simulink model "DAB_3phase_final"  (R2022b)
settings: Solver=ode23t  StartTime=0.0  StopTime=1/100000*10000  MaxStep=1/100000  RelTol=1e-3  AbsTol=1e-3
StartFcn:
  | tic
StopFcn:
  | toc
undefined symbols (not defined in the file): Vdc, Vth
libraries: nesl_utility x24, fl_lib x21, ee_lib x13, simulink x6, slpidlib x1
settings Model: SimulationMode=accelerator  Creator=jvansick  LastModifiedBy=jvansick
settings SolverCC: ExtrapolationOrder=1  ZeroCrossAlgorithm=Adaptive  ODENIntegrationMethod=ode14x
settings DebuggingCC: UnconnectedInputMsg=warning  UnconnectedOutputMsg=warning  UnconnectedLineMsg=warning
settings ModelReferenceCC: EnableRefExpFcnMdlSchedulingChecks=on
settings RTWCC: DLArmComputeVersion=19.05

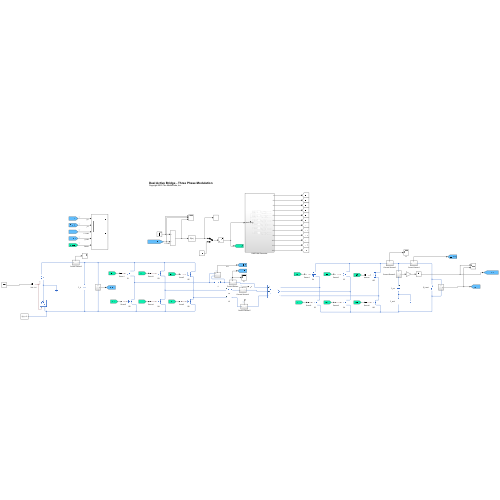
[thumbnail: Simulink's stored preview of the top-level diagram]
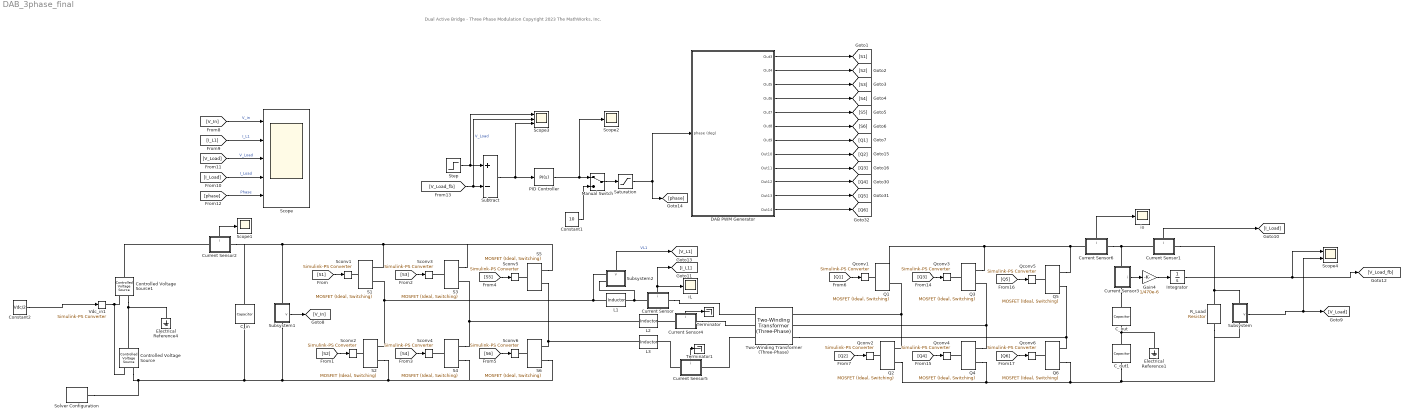
== system DAB_3phase_final ==
  note: Dual Active Bridge - Three Phase Modulation
      | Copyright 2023 The MathWorks, Inc.
  C_in : fl_lib/Electrical/Electrical Elements/Capacitor  c=220e-6 F  r=1e-6 Ohm  g=0 1/Ohm  i_specify=off  i_priority=None  i=0 A  i_nominal_specify=off  i_nominal_unit=A  i_nominal_value=1  v_specify=off  v_priority=None  v=0 V  v_nominal_specify=off  v_nominal_unit=V  v_nominal_value=1  vc_specify=on  vc_priority=High  vc=Vdc V  vc_nominal_specify=off  vc_nominal_unit=V  vc_nominal_value=1
  C_out : fl_lib/Electrical/Electrical Elements/Capacitor  c=(470e-6)*2 F  r=0 Ohm  g=0 1/Ohm  i_specify=off  i_priority=None  i=0 A  i_nominal_specify=off  i_nominal_unit=A  i_nominal_value=1  v_specify=off  v_priority=None  v=0 V  v_nominal_specify=off  v_nominal_unit=V  v_nominal_value=1  vc_specify=on  vc_priority=High  vc=200 V  vc_nominal_specify=off  vc_nominal_unit=V  vc_nominal_value=1
  C_out1 : fl_lib/Electrical/Electrical Elements/Capacitor  c=(470e-6)*2 F  r=0 Ohm  g=0 1/Ohm  i_specify=off  i_priority=None  i=0 A  i_nominal_specify=off  i_nominal_unit=A  i_nominal_value=1  v_specify=off  v_priority=None  v=0 V  v_nominal_specify=off  v_nominal_unit=V  v_nominal_value=1  vc_specify=on  vc_priority=High  vc=200 V  vc_nominal_specify=off  vc_nominal_unit=V  vc_nominal_value=1
  Constant1 : Constant  Value=10  SampleTime=-1
  Constant2 : Constant  Value=Vdc/2
  Controlled Voltage Source : fl_lib/Electrical/Electrical Sources/Controlled Voltage Source
  Controlled Voltage Source1 : fl_lib/Electrical/Electrical Sources/Controlled Voltage Source
  Current Sensor : Subsystem
      settings: PortSchema="{\"entries\":[{\"content\":{\"sides\":[{\"content\":{\"connectorIds\":[\"LConn1\"]},\"type\":\"ConnectorPlacement.EquallySpacedRectSide\",\"uuid\":\"e9388151-e471-4783-81c5-5134e1313d7c\"},{\"content\":{\"connectorIds\":[\"RConn1\"],\"side\":\"RIGHT\"},\"type\":\"ConnectorPlacement.EquallySpacedRectSide\",\"uuid\":\"bcb23f28-0826-4736-ab91-150a314eb643\"},{\"content\":{\"connectorIds\":[\"Out1\"],\"side\":\"TOP\"},\"type\":\"ConnectorPlacement.EquallySpacedRectSide\",\"uuid\":\"e1937689-3337-4922-a316-f56c73fb0974\"}]},\"type\":\"ConnectorPlacement.EquallySpacedConnector\",\"uuid\":\"dc34a384-5aa5-46fc-88a5-47651899efae\"}],\"packageUris\":[\"http://schema.mathworks.com/mf0/Connector/R2020b\"],\"version\":\"1.0\"}"
  Current Sensor1 : Subsystem
      settings: PortSchema="{\"entries\":[{\"content\":{\"sides\":[{\"content\":{\"connectorIds\":[\"LConn1\"]},\"type\":\"ConnectorPlacement.EquallySpacedRectSide\",\"uuid\":\"e9388151-e471-4783-81c5-5134e1313d7c\"},{\"content\":{\"connectorIds\":[\"RConn1\"],\"side\":\"RIGHT\"},\"type\":\"ConnectorPlacement.EquallySpacedRectSide\",\"uuid\":\"bcb23f28-0826-4736-ab91-150a314eb643\"},{\"content\":{\"connectorIds\":[\"Out1\"],\"side\":\"TOP\"},\"type\":\"ConnectorPlacement.EquallySpacedRectSide\",\"uuid\":\"e1937689-3337-4922-a316-f56c73fb0974\"}]},\"type\":\"ConnectorPlacement.EquallySpacedConnector\",\"uuid\":\"dc34a384-5aa5-46fc-88a5-47651899efae\"}],\"packageUris\":[\"http://schema.mathworks.com/mf0/Connector/R2020b\"],\"version\":\"1.0\"}"
  Current Sensor2 : Subsystem
      settings: PortSchema="{\"entries\":[{\"content\":{\"sides\":[{\"content\":{\"connectorIds\":[\"LConn1\"]},\"type\":\"ConnectorPlacement.EquallySpacedRectSide\",\"uuid\":\"e9388151-e471-4783-81c5-5134e1313d7c\"},{\"content\":{\"connectorIds\":[\"RConn1\"],\"side\":\"RIGHT\"},\"type\":\"ConnectorPlacement.EquallySpacedRectSide\",\"uuid\":\"bcb23f28-0826-4736-ab91-150a314eb643\"},{\"content\":{\"connectorIds\":[\"Out1\"],\"side\":\"TOP\"},\"type\":\"ConnectorPlacement.EquallySpacedRectSide\",\"uuid\":\"e1937689-3337-4922-a316-f56c73fb0974\"}]},\"type\":\"ConnectorPlacement.EquallySpacedConnector\",\"uuid\":\"dc34a384-5aa5-46fc-88a5-47651899efae\"}],\"packageUris\":[\"http://schema.mathworks.com/mf0/Connector/R2020b\"],\"version\":\"1.0\"}"
  Current Sensor3 : Subsystem
      settings: PortSchema="{\"entries\":[{\"content\":{\"sides\":[{\"content\":{\"connectorIds\":[\"LConn1\"]},\"type\":\"ConnectorPlacement.EquallySpacedRectSide\",\"uuid\":\"e9388151-e471-4783-81c5-5134e1313d7c\"},{\"content\":{\"connectorIds\":[\"RConn1\"],\"side\":\"RIGHT\"},\"type\":\"ConnectorPlacement.EquallySpacedRectSide\",\"uuid\":\"bcb23f28-0826-4736-ab91-150a314eb643\"},{\"content\":{\"connectorIds\":[\"Out1\"],\"side\":\"TOP\"},\"type\":\"ConnectorPlacement.EquallySpacedRectSide\",\"uuid\":\"e1937689-3337-4922-a316-f56c73fb0974\"}]},\"type\":\"ConnectorPlacement.EquallySpacedConnector\",\"uuid\":\"dc34a384-5aa5-46fc-88a5-47651899efae\"}],\"packageUris\":[\"http://schema.mathworks.com/mf0/Connector/R2020b\"],\"version\":\"1.0\"}"
  Current Sensor4 : Subsystem
      settings: PortSchema="{\"entries\":[{\"content\":{\"sides\":[{\"content\":{\"connectorIds\":[\"LConn1\"]},\"type\":\"ConnectorPlacement.EquallySpacedRectSide\",\"uuid\":\"e9388151-e471-4783-81c5-5134e1313d7c\"},{\"content\":{\"connectorIds\":[\"RConn1\"],\"side\":\"RIGHT\"},\"type\":\"ConnectorPlacement.EquallySpacedRectSide\",\"uuid\":\"bcb23f28-0826-4736-ab91-150a314eb643\"},{\"content\":{\"connectorIds\":[\"Out1\"],\"side\":\"TOP\"},\"type\":\"ConnectorPlacement.EquallySpacedRectSide\",\"uuid\":\"e1937689-3337-4922-a316-f56c73fb0974\"}]},\"type\":\"ConnectorPlacement.EquallySpacedConnector\",\"uuid\":\"dc34a384-5aa5-46fc-88a5-47651899efae\"}],\"packageUris\":[\"http://schema.mathworks.com/mf0/Connector/R2020b\"],\"version\":\"1.0\"}"
  Current Sensor5 : Subsystem
      settings: PortSchema="{\"entries\":[{\"content\":{\"sides\":[{\"content\":{\"connectorIds\":[\"LConn1\"]},\"type\":\"ConnectorPlacement.EquallySpacedRectSide\",\"uuid\":\"e9388151-e471-4783-81c5-5134e1313d7c\"},{\"content\":{\"connectorIds\":[\"RConn1\"],\"side\":\"RIGHT\"},\"type\":\"ConnectorPlacement.EquallySpacedRectSide\",\"uuid\":\"bcb23f28-0826-4736-ab91-150a314eb643\"},{\"content\":{\"connectorIds\":[\"Out1\"],\"side\":\"TOP\"},\"type\":\"ConnectorPlacement.EquallySpacedRectSide\",\"uuid\":\"e1937689-3337-4922-a316-f56c73fb0974\"}]},\"type\":\"ConnectorPlacement.EquallySpacedConnector\",\"uuid\":\"dc34a384-5aa5-46fc-88a5-47651899efae\"}],\"packageUris\":[\"http://schema.mathworks.com/mf0/Connector/R2020b\"],\"version\":\"1.0\"}"
  Current Sensor6 : Subsystem
      settings: PortSchema="{\"entries\":[{\"content\":{\"sides\":[{\"content\":{\"connectorIds\":[\"LConn1\"]},\"type\":\"ConnectorPlacement.EquallySpacedRectSide\",\"uuid\":\"e9388151-e471-4783-81c5-5134e1313d7c\"},{\"content\":{\"connectorIds\":[\"RConn1\"],\"side\":\"RIGHT\"},\"type\":\"ConnectorPlacement.EquallySpacedRectSide\",\"uuid\":\"bcb23f28-0826-4736-ab91-150a314eb643\"},{\"content\":{\"connectorIds\":[\"Out1\"],\"side\":\"TOP\"},\"type\":\"ConnectorPlacement.EquallySpacedRectSide\",\"uuid\":\"e1937689-3337-4922-a316-f56c73fb0974\"}]},\"type\":\"ConnectorPlacement.EquallySpacedConnector\",\"uuid\":\"dc34a384-5aa5-46fc-88a5-47651899efae\"}],\"packageUris\":[\"http://schema.mathworks.com/mf0/Connector/R2020b\"],\"version\":\"1.0\"}"
  DAB PWM Generator : Subsystem
  Electrical Reference1 : fl_lib/Electrical/Electrical Elements/Electrical Reference
  Electrical Reference4 : fl_lib/Electrical/Electrical Elements/Electrical Reference
  Gain4 : Gain  Gain=1/470e-6
  Integrator : Integrator  InitialCondition=400
  L1 : fl_lib/Electrical/Electrical Elements/Inductor  l=36e-6 H  r=0.01 Ohm  g=1e-6 1/Ohm  i_specify=off  i_priority=None  i=0 A  i_nominal_specify=off  i_nominal_unit=A  i_nominal_value=1  v_specify=off  v_priority=None  v=0 V  v_nominal_specify=off  v_nominal_unit=V  v_nominal_value=1  i_L_specify=off  i_L_priority=High  i_L=0 A  i_L_nominal_specify=off  i_L_nominal_unit=A  i_L_nominal_value=1
  L2 : fl_lib/Electrical/Electrical Elements/Inductor  l=36e-6 H  r=0.01 Ohm  g=1e-6 1/Ohm  i_specify=off  i_priority=None  i=0 A  i_nominal_specify=off  i_nominal_unit=A  i_nominal_value=1  v_specify=off  v_priority=None  v=0 V  v_nominal_specify=off  v_nominal_unit=V  v_nominal_value=1  i_L_specify=off  i_L_priority=High  i_L=0 A  i_L_nominal_specify=off  i_L_nominal_unit=A  i_L_nominal_value=1
  L3 : fl_lib/Electrical/Electrical Elements/Inductor  l=36e-6 H  r=0.01 Ohm  g=1e-6 1/Ohm  i_specify=off  i_priority=None  i=0 A  i_nominal_specify=off  i_nominal_unit=A  i_nominal_value=1  v_specify=off  v_priority=None  v=0 V  v_nominal_specify=off  v_nominal_unit=V  v_nominal_value=1  i_L_specify=off  i_L_priority=High  i_L=0 A  i_L_nominal_specify=off  i_L_nominal_unit=A  i_L_nominal_value=1
  Manual Switch : ManualSwitch
  PID Controller : slpidlib/PID Controller  Controller=PI  Form=Parallel  TimeDomain=Continuous-time  UseExternalTs=off  SampleTime=-1  IntegratorMethod=Forward Euler  FilterMethod=Forward Euler  ControllerParametersSource=internal  P=0.3  I=60  UseKiTs=off  D=0  N=100  UseFilter=on  TunerSelectOption=Transfer Function Based (PID Tuner App)  InitialConditionSource=internal  InitialConditionForIntegrator=0  InitialConditionForFilter=0  DifferentiatorICPrevScaledInput=0  ExternalReset=none  TrackingMode=off  Kt=1  LimitOutput=off  SatLimitsSource=internal  UpperSaturationLimit=inf  LowerSaturationLimit=-inf  LinearizeAsGain=on  AntiWindupMode=none  Kb=1  LimitIntegrator=off  UpperIntegratorSaturationLimit=inf  LowerIntegratorSaturationLimit=-inf  POutMin=[]  POutMax=[]  IOutMin=[]  IOutMax=[]  DOutMin=[]  DOutMax=[]  NOutMin=[]  NOutMax=[]  SumOutMin=[]  SumOutMax=[]  SaturationOutMin=[]  SaturationOutMax=[]  PParamMin=[]  PParamMax=[]  IParamMin=[]  IParamMax=[]  DParamMin=[]  DParamMax=[]  NParamMin=[]  NParamMax=[]  KbParamMin=[]  KbParamMax=[]  KtParamMin=[]  KtParamMax=[]  KbOutMin=[]  KbOutMax=[]  KtOutMin=[]  KtOutMax=[]  IntegratorOutMin=[]  IntegratorOutMax=[]  FilterOutMin=[]  FilterOutMax=[]  SumI1OutMin=[]  SumI1OutMax=[]  SumI2OutMin=[]  SumI2OutMax=[]  SumI3OutMin=[]  SumI3OutMax=[]  SumI4OutMin=[]  SumI4OutMax=[]  SumDOutMin=[]  SumDOutMax=[]  DifferentiatorOutMin=[]  DifferentiatorOutMax=[]  FilterDiffOutCoefMin=[]  FilterDiffOutCoefMax=[]  ReciprocalOutMin=[]  ReciprocalOutMax=[]  SumDenOutMin=[]  SumDenOutMax=[]  SumNumOutMin=[]  SumNumOutMax=[]  DivideOutMin=[]  DivideOutMax=[]  UdiffTsProdOutMin=[]  UdiffTsProdOutMax=[]  NTsProdOutMin=[]  NTsProdOutMax=[]  UintegralTsProdOutMin=[]  UintegralTsProdOutMax=[]  UngainTsProdOutMin=[]  UngainTsProdOutMax=[]  ClampingZeroOutDataTypeStr=Inherit: Inherit via back propagation  ClampingZeroOutMin=[]  ClampingZeroOutMax=[]  FilterDenConstantOutDataTypeStr=Inherit: Inherit via back propagation  FilterDenConstantOutMin=[]  FilterDenConstantOutMax=[]  PCopyOutDataTypeStr=Inherit: Inherit via back propagation  PCopyOutMin=[]  PCopyOutMax=[]  NCopyOutDataTypeStr=Inherit: Inherit via back propagation  NCopyOutMin=[]  NCopyOutMax=[]  IntegratorContinuousStateAttributes=''  IntegratorStateMustResolveToSignalObject=off  IntegratorRTWStateStorageClass=Auto  FilterContinuousStateAttributes=''  FilterStateMustResolveToSignalObject=off  FilterRTWStateStorageClass=Auto  ParallelPVariant=InternalParameters  IdealPVariant=Disabled  IVariant=InternalParameters  DVariant=Disabled  IntegratorVariant=Continuous  SatVariant=Disabled  AWVariant=Passthrough  PCopyVariant=Disabled  TRVariant=Disabled  FdbkBlocksVariant=Forward  IdealPFdbkVariant=Disabled  SatFdbkVariant=Disabled  DerivativeFilterVariant=Disabled  NVariant=Disabled  NCopyVariant=Disabled_SignalSpec  FilterICVariant=Disabled  IntegratorICVariant=InternalICs  ExternalResetVariant=Disabled  TRSumVariant=Passthrough  SumFdbkVariant=Disabled  SumVariant=Sum_PI  TsampFilterVariant=InternalTs  TsampNgainVariant=Passthrough  TsampIntegralVariant=Passthrough  ExternalSaturationOutDataTypeStr=Inherit: Same as second input
  Q{1..6} (6 alike) : ee_lib/Semiconductors & Converters/MOSFET (Ideal, Switching)  port_option=ee.enum.controlport.ps  Rds=R_ds Ohm  Goff=1e-5 1/Ohm  Vth=Vth V  diode_param=2  diode_Vf=0.8 V  diode_Ron=0.001 Ohm  diode_Goff=1e-5 1/Ohm  diode_C=50e-9 F  diode_iRM=-235 A  diode_iF=300 A  diode_idot=-50 A/us  diode_trr_param=1  diode_trr_factor=3  diode_trr=15 us  diode_Qrr=1500 s*uA  ids_specify=off  ids_priority=None  ids=0 A  ids_nominal_specify=off  ids_nominal_unit=A  ids_nominal_value=1  vds_specify=off  vds_priority=None  vds=0 V  vds_nominal_specify=off  vds_nominal_unit=V  vds_nominal_value=1  vgs_specify=off  vgs_priority=None  vgs=0 V  vgs_nominal_specify=off  vgs_nominal_unit=V  vgs_nominal_value=1  thermal_loss_option=ee.enum.converters.thermalLossOption.constantvalues  Von_data=[0, 1.8, 3.2, 6, 10, 16; 0, 2, 5.5, 9.5, 15, 25] V  Tj=[298.15, 448.15] K  Iout_data=[0, 20, 40, 60, 80, 100] A  Eon_data=[0, 55.04, 124.57, 235.53, 362.12; 0, 71.25, 161.25, 304.88, 468.75] * 1e-6 J  Eoff_data=[0, 18, 30, 56.1, 76.5; 0, 22.5, 37.5, 70.13, 95.63] * 1e-6 J  Tj_loss=[298.15, 448.15] K  Iout_data_loss=[0, 10, 20, 30, 40] A  Eon_scalar=22.86e-3 J  Eoff_scalar=17.14e-3 J  Voff=300 V  Iout_scalar=600 A  diodeModelType=ee.enum.converters.diodeModelType.pwl  diodeTableType=ee.enum.diode.tableType.IfMat  diode_IfMat=[.07, .12, .19, 1.75, 4.24, 7.32, 11.2; .16, .3, .72, 2.14, 4.02, 6.35, 9.12] A  diode_VfMat=[.9, 1.15, 1.25, 1.5, 1.75, 2.17, 2.6, 2.85; .58, .68, .75, 1.1, 1.38, 1.77, 2.27, 2.7] V  diode_TjVec=[25, 125] degC  diode_VfVec=[.5, .7, .9, 1.3, 1.7, 2.1, 2.5] V  diode_IfVec=[.1, .2, .5, 1, 2, 4, 7, 10] A  diode_Vr=-600 V  diode_Ls=150 nH  diode_Erec=0.03 J  thermal_network_parameterization=ee.enum.thermalNetworkTopology.external  Rth=[.03, .2] K/W  Rth_Cauer=[.03, .1, .2] K/W  Rth_Foster=[.03, .2] K/W  thermal_mass_parameterization=ee.enum.thermalNetwork.timeconstant  thermal_mass=[3, 25] J/K  thermal_mass_Cauer=[3, 10, 25] J/K  thermal_mass_Foster=[33, 50] J/K  thermal_time_constant=[.1, 5] s  thermal_time_constant_Cauer=[.1, 1, 5] s  thermal_time_constant_Foster=[1, 10] s  thermal_mass_initial_temperatures=[25, 25] degC  thermal_mass_initial_temperatures_Cauer=[25, 25, 25] degC  junction_thermal_mass=0.1 J/K  Tvec_initial_Foster=[25, 25, 25, 25] degC  no_thermal_network=0  junction_temperature_specify=off  junction_temperature_priority=None  junction_temperature=25 degC  junction_temperature_nominal_specify=off  junction_temperature_nominal_unit=degC  junction_temperature_nominal_value=1  Qj_specify=off  Qj_priority=None  Qj=0 W  Qj_nominal_specify=off  Qj_nominal_unit=W  Qj_nominal_value=1
  Qconv{1..6} (6 alike) : nesl_utility/Simulink-PS Converter  PhysicalDomain=network_engine_domain  SubClassName=ps_input  LeftPortType=input  RightPortType=output  PseudoPeriodic=off  Frequencies=[]  NoiseDistribution=none  NoiseParameters=[]  Unit=1  AffineConversion=off  FilteringAndDerivatives=provide  SimscapeFilterOrder=1  InputFilterTimeConstant=0.001  UdotUserProvided=0
  R_Load : fl_lib/Electrical/Electrical Elements/Resistor  R=26 Ohm  i_specify=off  i_priority=None  i=0 A  i_nominal_specify=off  i_nominal_unit=A  i_nominal_value=1  v_specify=off  v_priority=None  v=0 V  v_nominal_specify=off  v_nominal_unit=V  v_nominal_value=1
  S{1..6} (6 alike) : ee_lib/Semiconductors & Converters/MOSFET (Ideal, Switching)  port_option=ee.enum.controlport.ps  Rds=R_ds Ohm  Goff=1e-5 1/Ohm  Vth=Vth V  diode_param=2  diode_Vf=0.8 V  diode_Ron=0.001 Ohm  diode_Goff=1e-5 1/Ohm  diode_C=50e-9 F  diode_iRM=-235 A  diode_iF=300 A  diode_idot=-50 A/us  diode_trr_param=1  diode_trr_factor=3  diode_trr=15 us  diode_Qrr=1500 s*uA  ids_specify=off  ids_priority=None  ids=0 A  ids_nominal_specify=off  ids_nominal_unit=A  ids_nominal_value=1  vds_specify=off  vds_priority=None  vds=0 V  vds_nominal_specify=off  vds_nominal_unit=V  vds_nominal_value=1  vgs_specify=off  vgs_priority=None  vgs=0 V  vgs_nominal_specify=off  vgs_nominal_unit=V  vgs_nominal_value=1  thermal_loss_option=ee.enum.converters.thermalLossOption.constantvalues  Von_data=[0, 1.8, 3.2, 6, 10, 16; 0, 2, 5.5, 9.5, 15, 25] V  Tj=[298.15, 448.15] K  Iout_data=[0, 20, 40, 60, 80, 100] A  Eon_data=[0, 55.04, 124.57, 235.53, 362.12; 0, 71.25, 161.25, 304.88, 468.75] * 1e-6 J  Eoff_data=[0, 18, 30, 56.1, 76.5; 0, 22.5, 37.5, 70.13, 95.63] * 1e-6 J  Tj_loss=[298.15, 448.15] K  Iout_data_loss=[0, 10, 20, 30, 40] A  Eon_scalar=22.86e-3 J  Eoff_scalar=17.14e-3 J  Voff=300 V  Iout_scalar=600 A  diodeModelType=ee.enum.converters.diodeModelType.pwl  diodeTableType=ee.enum.diode.tableType.IfMat  diode_IfMat=[.07, .12, .19, 1.75, 4.24, 7.32, 11.2; .16, .3, .72, 2.14, 4.02, 6.35, 9.12] A  diode_VfMat=[.9, 1.15, 1.25, 1.5, 1.75, 2.17, 2.6, 2.85; .58, .68, .75, 1.1, 1.38, 1.77, 2.27, 2.7] V  diode_TjVec=[25, 125] degC  diode_VfVec=[.5, .7, .9, 1.3, 1.7, 2.1, 2.5] V  diode_IfVec=[.1, .2, .5, 1, 2, 4, 7, 10] A  diode_Vr=-600 V  diode_Ls=150 nH  diode_Erec=0.03 J  thermal_network_parameterization=ee.enum.thermalNetworkTopology.external  Rth=[.03, .2] K/W  Rth_Cauer=[.03, .1, .2] K/W  Rth_Foster=[.03, .2] K/W  thermal_mass_parameterization=ee.enum.thermalNetwork.timeconstant  thermal_mass=[3, 25] J/K  thermal_mass_Cauer=[3, 10, 25] J/K  thermal_mass_Foster=[33, 50] J/K  thermal_time_constant=[.1, 5] s  thermal_time_constant_Cauer=[.1, 1, 5] s  thermal_time_constant_Foster=[1, 10] s  thermal_mass_initial_temperatures=[25, 25] degC  thermal_mass_initial_temperatures_Cauer=[25, 25, 25] degC  junction_thermal_mass=0.1 J/K  Tvec_initial_Foster=[25, 25, 25, 25] degC  no_thermal_network=0  junction_temperature_specify=off  junction_temperature_priority=None  junction_temperature=25 degC  junction_temperature_nominal_specify=off  junction_temperature_nominal_unit=degC  junction_temperature_nominal_value=1  Qj_specify=off  Qj_priority=None  Qj=0 W  Qj_nominal_specify=off  Qj_nominal_unit=W  Qj_nominal_value=1
  Saturation : Saturate  UpperLimit=180  LowerLimit=0
  Sconv{1..6} (6 alike) : nesl_utility/Simulink-PS Converter  PhysicalDomain=network_engine_domain  SubClassName=ps_input  LeftPortType=input  RightPortType=output  PseudoPeriodic=off  Frequencies=[]  NoiseDistribution=none  NoiseParameters=[]  Unit=1  AffineConversion=off  FilteringAndDerivatives=provide  SimscapeFilterOrder=1  InputFilterTimeConstant=0.001  UdotUserProvided=0
  Scope : Scope  NumInputPorts=5
  Scope1 : Scope
  Scope2 : Scope
  Scope3 : Scope  NumInputPorts=3
  Scope4 : Scope  NumInputPorts=2
  Solver Configuration : nesl_utility/Solver Configuration  PhysicalDomain=network_engine_domain  SubClassName=solver  LeftPortType=input  RightPortType=generic  Tones=[]  Harmonics=[]  SimulateNoise=off  Profile=off  UseLocalSampling=off  EnableSwitchedLinearOptims=on  FrequencyDomain=off  UseCCode=off  RelTol=0.001  AbsTol=1e-06  MinStep=1e-09  ToWorkspace=off  RevertToSquareIcSolve=off  NumHomotopyIterations=100  PhasorMode=off  PhasorModeNumHarmonics=1  ConsistencySolver=NEWTON_FTOL  IndexReductionMethod=DerivativeReplacement  DoDC=off  ResidualTolerance=1e-09  ConsistencyTolSource=GLOBAL  ConsistencyAbsTol=0.001  ConsistencyRelTol=0.001  ConsistencyTolFactor=0.001  UseLocalSolver=off  LocalSolverChoice=NE_BACKWARD_EULER_ADVANCER  ResolveIndetEquations=on  FunctionEvalNumThread=1  LocalSolverSampleTime=1/100000/100  DoFixedCost=off  MaxNonlinIter=3  MaxModeIter=2  ComputeImpulses=off  ImpulseIterations=2  LinearAlgebra=auto  LinearAlgebraNumThread=0  EquationFormulation=NE_TIME_EF  DelaysMemoryBudget=1024  AutomaticFiltering=on  FilteringTimeConstant=0.001  PartitionStorageMethod=AS_NEEDED  PartitionMemoryBudget=1024  PartitionMethod=ROBUST
  Step : Step  Time=1/100000*10000/2  Before=400  After=500  SampleTime=0
  Subsystem : Subsystem
      settings: PortSchema="{\"entries\":[{\"content\":{\"sides\":[{\"content\":{\"connectorIds\":[\"LConn1\"]},\"type\":\"ConnectorPlacement.EquallySpacedRectSide\",\"uuid\":\"e9388151-e471-4783-81c5-5134e1313d7c\"},{\"content\":{\"connectorIds\":[\"RConn1\"],\"side\":\"RIGHT\"},\"type\":\"ConnectorPlacement.EquallySpacedRectSide\",\"uuid\":\"bcb23f28-0826-4736-ab91-150a314eb643\"},{\"content\":{\"connectorIds\":[\"Out1\"],\"side\":\"TOP\"},\"type\":\"ConnectorPlacement.EquallySpacedRectSide\",\"uuid\":\"e1937689-3337-4922-a316-f56c73fb0974\"}]},\"type\":\"ConnectorPlacement.EquallySpacedConnector\",\"uuid\":\"dc34a384-5aa5-46fc-88a5-47651899efae\"}],\"packageUris\":[\"http://schema.mathworks.com/mf0/Connector/R2020b\"],\"version\":\"1.0\"}"
  Subsystem1 : Subsystem
      settings: PortSchema="{\"entries\":[{\"content\":{\"sides\":[{\"content\":{\"connectorIds\":[\"LConn1\"]},\"type\":\"ConnectorPlacement.EquallySpacedRectSide\",\"uuid\":\"e9388151-e471-4783-81c5-5134e1313d7c\"},{\"content\":{\"connectorIds\":[\"RConn1\"],\"side\":\"RIGHT\"},\"type\":\"ConnectorPlacement.EquallySpacedRectSide\",\"uuid\":\"bcb23f28-0826-4736-ab91-150a314eb643\"},{\"content\":{\"connectorIds\":[\"Out1\"],\"side\":\"TOP\"},\"type\":\"ConnectorPlacement.EquallySpacedRectSide\",\"uuid\":\"e1937689-3337-4922-a316-f56c73fb0974\"}]},\"type\":\"ConnectorPlacement.EquallySpacedConnector\",\"uuid\":\"dc34a384-5aa5-46fc-88a5-47651899efae\"}],\"packageUris\":[\"http://schema.mathworks.com/mf0/Connector/R2020b\"],\"version\":\"1.0\"}"
  Subsystem2 : Subsystem
      settings: PortSchema="{\"entries\":[{\"content\":{\"sides\":[{\"content\":{\"connectorIds\":[\"LConn1\",\"LConn2\"]},\"type\":\"ConnectorPlacement.EquallySpacedRectSide\",\"uuid\":\"e9388151-e471-4783-81c5-5134e1313d7c\"},{\"content\":{\"connectorIds\":[],\"side\":\"RIGHT\"},\"type\":\"ConnectorPlacement.EquallySpacedRectSide\",\"uuid\":\"bcb23f28-0826-4736-ab91-150a314eb643\"},{\"content\":{\"connectorIds\":[\"Out1\"],\"side\":\"TOP\"},\"type\":\"ConnectorPlacement.EquallySpacedRectSide\",\"uuid\":\"e1937689-3337-4922-a316-f56c73fb0974\"}]},\"type\":\"ConnectorPlacement.EquallySpacedConnector\",\"uuid\":\"dc34a384-5aa5-46fc-88a5-47651899efae\"}],\"packageUris\":[\"http://schema.mathworks.com/mf0/Connector/R2020b\"],\"version\":\"1.0\"}"
  Subtract : Sum  Inputs=+-
  Terminator : Terminator
  Terminator1 : Terminator
  Two-Winding Transformer (Three-Phase) : ee_lib/Passive/Transformers/Two-Winding Transformer (Three-Phase)  SRated=25e3 A*V  FRated=100000 Hz  Winding1Connection=ee.enum.windingconnection.Yg  VRated1=800 V  Winding2Connection=ee.enum.windingconnection.Yg  VRated2=500 V  CoreType=ee.enum.coretype.threelimb  pu_Rw1=0.01  pu_Rw2=0.01  leakage_reactance_option=ee.enum.transformer_leakage.exclude  pu_Xl1=0.05  pu_Xl2=0.05  magnetizing_resistance_option=ee.enum.transformer_magnetizingResistance.exclude  pu_Rm=500  magnetizing_reactance_option=ee.enum.transformer_magnetizingReactance.exclude  saturation_option=ee.enum.transformer_saturation.exclude  pu_Xm=500  current_data=[0, .002, 1, 2]  magnetic_flux_data=[0, 1.2, 1.5, 1.51]  pu_X0=0.5  i1_specify=off  i1_priority=None  i1=[0, 0, 0] A  i1_nominal_specify=off  i1_nominal_unit=A  i1_nominal_value=1  i2_specify=off  i2_priority=None  i2=[0, 0, 0] A  i2_nominal_specify=off  i2_nominal_unit=A  i2_nominal_value=1  phi_specify=off  phi_priority=None  phi=[0, 0, 0]  phi_nominal_specify=off  phi_nominal_unit=1  phi_nominal_value=1  power_dissipated_specify=off  power_dissipated_priority=None  power_dissipated=0 W  power_dissipated_nominal_specify=off  power_dissipated_nominal_unit=W  power_dissipated_nominal_value=1
      settings: InternalSimscapePortConfiguration="{\"Bottom\":[],\"Left\":[{\"id\":\"a1\",\"label\":\"a1\",\"type\":\"foundation.electrical.electrical\"},{\"id\":\"b1\",\"label\":\"b1\",\"type\":\"foundation.electrical.electrical\"},{\"id\":\"c1\",\"label\":\"c1\",\"type\":\"foundation.electrical.electrical\"}],\"Right\":[{\"id\":\"a2\",\"label\":\"a2\",\"type\":\"foundation.electrical.electrical\"},{\"id\":\"b2\",\"label\":\"b2\",\"type\":\"foundation.electrical.electrical\"},{\"id\":\"c2\",\"label\":\"c2\",\"type\":\"foundation.electrical.electrical\"}],\"Top\":[]}"
  Vdc_in1 : nesl_utility/Simulink-PS Converter  PhysicalDomain=network_engine_domain  SubClassName=ps_input  LeftPortType=input  RightPortType=output  PseudoPeriodic=off  Frequencies=[]  NoiseDistribution=none  NoiseParameters=[]  Unit=1  AffineConversion=off  FilteringAndDerivatives=provide  SimscapeFilterOrder=1  InputFilterTimeConstant=0.001  UdotUserProvided=0
  iL : Scope
  io : Scope
  wires:
  [S1] -> Sconv1/1
  [S2] -> Sconv2/1
  [S3] -> Sconv3/1
  [S4] -> Sconv4/1
  Subsystem1/1(v) -> [V_In]
  Subsystem/1(v) -> Scope4/2, [V_Load]
  Current Sensor1/1(i) -> [I_Load]
  Current Sensor/1(i) -> [I_L1], iL/1
  [V_In] -> Scope/1  "V_in"
  [I_L1] -> Scope/2  "I_L1"
  [I_Load] -> Scope/4  "I_Load"
  [V_Load] -> Scope/3  "V_Load"
  Current Sensor2/1(i) -> Scope1/1
  Current Sensor3/1(i) -> Gain4/1
  Integrator/1 -> Scope4/1, [V_Load_fb]
  Subsystem2/1(v) -> [V_L1]  "VL1"
  [phase] -> Scope/5  "Phase"
  [S6] -> Sconv6/1
  [S5] -> Sconv5/1
  [Q5] -> Qconv5/1
  [Q6] -> Qconv6/1
  [Q3] -> Qconv3/1
  [Q1] -> Qconv1/1
  [Q4] -> Qconv4/1
  [Q2] -> Qconv2/1
  Subtract/1 -> Scope3/3, PID Controller/1
  [V_Load_fb] -> Scope3/2, Subtract/2  "V_Load"
  Step/1 -> Scope3/1, Subtract/1
  Saturation/1 -> [phase], DAB PWM Generator/1(phase (deg))
  Current Sensor4/1(i) -> Terminator/1
  DAB PWM Generator/1(Out3) -> [S1]
  DAB PWM Generator/2(Out4) -> [S2]
  DAB PWM Generator/3(Out5) -> [S3]
  DAB PWM Generator/4(Out6) -> [S4]
  DAB PWM Generator/5(Out7) -> [S5]
  DAB PWM Generator/6(Out8) -> [S6]
  Current Sensor5/1(i) -> Terminator1/1
  DAB PWM Generator/7(Out9) -> [Q1]
  DAB PWM Generator/8(Out10) -> [Q2]
  DAB PWM Generator/9(Out11) -> [Q3]
  DAB PWM Generator/10(Out12) -> [Q4]
  DAB PWM Generator/11(Out13) -> [Q5]
  DAB PWM Generator/12(Out14) -> [Q6]
  Current Sensor6/1(i) -> io/1
  PID Controller/1 -> Scope2/1, Manual Switch/1
  Manual Switch/1 -> Saturation/1
  Constant1/1 -> Manual Switch/2
  Constant2/1 -> Vdc_in1/1
  Gain4/1 -> Integrator/1
  connections:
  Subsystem1/LConn1 -- Current Sensor2/RConn1 -- C_in/LConn1 -- S5/RConn1 -- S3/RConn1 -- S1/RConn1
  Controlled Voltage Source/RConn2 -- Solver Configuration/RConn1 -- Subsystem1/RConn1 -- S6/RConn2 -- S4/RConn2 -- S2/RConn2 -- C_in/RConn1
  S2/LConn1 -- Sconv2/RConn1
  Sconv1/RConn1 -- S1/LConn1
  S3/LConn1 -- Sconv3/RConn1
  S4/LConn1 -- Sconv4/RConn1
  Subsystem2/LConn1 -- S1/RConn2 -- S2/RConn1 -- L1/LConn1
  S4/RConn1 -- L2/LConn1 -- S3/RConn2
  R_Load/LConn1 -- Current Sensor1/RConn1 -- Subsystem/LConn1
  Current Sensor/LConn1 -- Subsystem2/LConn2 -- L1/RConn1
  Current Sensor3/RConn1 -- C_out/LConn1
  S5/RConn2 -- L3/LConn1 -- S6/RConn1
  S6/LConn1 -- Sconv6/RConn1
  S5/LConn1 -- Sconv5/RConn1
  Subsystem/RConn1 -- R_Load/RConn1 -- C_out1/RConn1 -- Q2/RConn2 -- Q4/RConn2 -- Q6/RConn2
  Current Sensor3/LConn1 -- Current Sensor6/RConn1 -- Current Sensor1/LConn1
  Q6/LConn1 -- Qconv6/RConn1
  Q3/LConn1 -- Qconv3/RConn1
  Q5/RConn2 -- Q6/RConn1 -- Two-Winding Transformer (Three-Phase)/RConn3
  Q2/RConn1 -- Q1/RConn2 -- Two-Winding Transformer (Three-Phase)/RConn1
  Q2/LConn1 -- Qconv2/RConn1
  Q4/LConn1 -- Qconv4/RConn1
  Q5/LConn1 -- Qconv5/RConn1
  Q4/RConn1 -- Q3/RConn2 -- Two-Winding Transformer (Three-Phase)/RConn2
  Qconv1/RConn1 -- Q1/LConn1
  Current Sensor4/LConn1 -- L2/RConn1
  Current Sensor5/LConn1 -- L3/RConn1
  Two-Winding Transformer (Three-Phase)/LConn3 -- Current Sensor5/RConn1
  Q5/RConn1 -- Current Sensor6/LConn1 -- Q1/RConn1 -- Q3/RConn1
  C_out1/LConn1 -- Electrical Reference1/LConn1 -- C_out/RConn1
  Vdc_in1/RConn1 -- Controlled Voltage Source1/RConn1 -- Controlled Voltage Source/RConn1
  Current Sensor2/LConn1 -- Controlled Voltage Source1/LConn1
  Controlled Voltage Source1/RConn2 -- Electrical Reference4/LConn1 -- Controlled Voltage Source/LConn1
  Current Sensor4/RConn1 -- Two-Winding Transformer (Three-Phase)/LConn2
  Current Sensor/RConn1 -- Two-Winding Transformer (Three-Phase)/LConn1

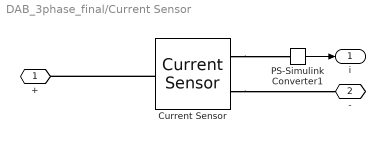
== system DAB_3phase_final/Current Sensor ==
  Current Sensor : fl_lib/Electrical/Electrical Sensors/Current Sensor
  PS-Simulink Converter1 : nesl_utility/PS-Simulink Converter  PhysicalDomain=network_engine_domain  SubClassName=ps_output  LeftPortType=input  RightPortType=output  PseudoPeriodic=off  Frequencies=[]  VectorFormat=1-D array  Unit=inherit  AffineConversion=off
  + : PMIOPort  Side=Left
  - : PMIOPort  Port=2  Side=Right
  i : Outport
  wires:
  PS-Simulink Converter1/1 -> i/1
  connections:
  Current Sensor/RConn1 -- PS-Simulink Converter1/LConn1
  Current Sensor/LConn1 -- +/RConn1
  Current Sensor/RConn2 -- -/RConn1

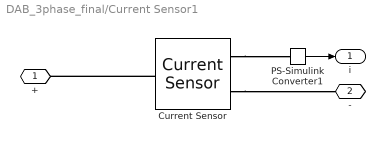
== system DAB_3phase_final/Current Sensor1 ==
  Current Sensor : fl_lib/Electrical/Electrical Sensors/Current Sensor
  PS-Simulink Converter1 : nesl_utility/PS-Simulink Converter  PhysicalDomain=network_engine_domain  SubClassName=ps_output  LeftPortType=input  RightPortType=output  PseudoPeriodic=off  Frequencies=[]  VectorFormat=1-D array  Unit=inherit  AffineConversion=off
  + : PMIOPort  Side=Left
  - : PMIOPort  Port=2  Side=Right
  i : Outport
  wires:
  PS-Simulink Converter1/1 -> i/1
  connections:
  Current Sensor/RConn2 -- -/RConn1
  Current Sensor/LConn1 -- +/RConn1
  Current Sensor/RConn1 -- PS-Simulink Converter1/LConn1

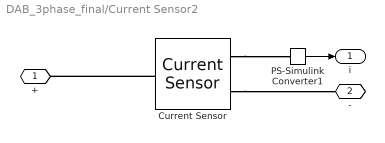
== system DAB_3phase_final/Current Sensor2 ==
  Current Sensor : fl_lib/Electrical/Electrical Sensors/Current Sensor
  PS-Simulink Converter1 : nesl_utility/PS-Simulink Converter  PhysicalDomain=network_engine_domain  SubClassName=ps_output  LeftPortType=input  RightPortType=output  PseudoPeriodic=off  Frequencies=[]  VectorFormat=1-D array  Unit=inherit  AffineConversion=off
  + : PMIOPort  Side=Left
  - : PMIOPort  Port=2  Side=Right
  i : Outport
  wires:
  PS-Simulink Converter1/1 -> i/1
  connections:
  Current Sensor/RConn2 -- -/RConn1
  Current Sensor/LConn1 -- +/RConn1
  Current Sensor/RConn1 -- PS-Simulink Converter1/LConn1

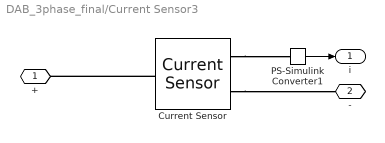
== system DAB_3phase_final/Current Sensor3 ==
  Current Sensor : fl_lib/Electrical/Electrical Sensors/Current Sensor
  PS-Simulink Converter1 : nesl_utility/PS-Simulink Converter  PhysicalDomain=network_engine_domain  SubClassName=ps_output  LeftPortType=input  RightPortType=output  PseudoPeriodic=off  Frequencies=[]  VectorFormat=1-D array  Unit=inherit  AffineConversion=off
  + : PMIOPort  Side=Left
  - : PMIOPort  Port=2  Side=Right
  i : Outport
  wires:
  PS-Simulink Converter1/1 -> i/1
  connections:
  Current Sensor/RConn1 -- PS-Simulink Converter1/LConn1
  Current Sensor/LConn1 -- +/RConn1
  Current Sensor/RConn2 -- -/RConn1

== system DAB_3phase_final/Current Sensor4 ==
  Current Sensor : fl_lib/Electrical/Electrical Sensors/Current Sensor
  PS-Simulink Converter1 : nesl_utility/PS-Simulink Converter  PhysicalDomain=network_engine_domain  SubClassName=ps_output  LeftPortType=input  RightPortType=output  PseudoPeriodic=off  Frequencies=[]  VectorFormat=1-D array  Unit=inherit  AffineConversion=off
  + : PMIOPort  Side=Left
  - : PMIOPort  Port=2  Side=Right
  i : Outport
  wires:
  PS-Simulink Converter1/1 -> i/1
  connections:
  Current Sensor/RConn1 -- PS-Simulink Converter1/LConn1
  Current Sensor/LConn1 -- +/RConn1
  Current Sensor/RConn2 -- -/RConn1

== system DAB_3phase_final/Current Sensor5 ==
  Current Sensor : fl_lib/Electrical/Electrical Sensors/Current Sensor
  PS-Simulink Converter1 : nesl_utility/PS-Simulink Converter  PhysicalDomain=network_engine_domain  SubClassName=ps_output  LeftPortType=input  RightPortType=output  PseudoPeriodic=off  Frequencies=[]  VectorFormat=1-D array  Unit=inherit  AffineConversion=off
  + : PMIOPort  Side=Left
  - : PMIOPort  Port=2  Side=Right
  i : Outport
  wires:
  PS-Simulink Converter1/1 -> i/1
  connections:
  Current Sensor/RConn1 -- PS-Simulink Converter1/LConn1
  Current Sensor/LConn1 -- +/RConn1
  Current Sensor/RConn2 -- -/RConn1

== system DAB_3phase_final/Current Sensor6 ==
  Current Sensor : fl_lib/Electrical/Electrical Sensors/Current Sensor
  PS-Simulink Converter1 : nesl_utility/PS-Simulink Converter  PhysicalDomain=network_engine_domain  SubClassName=ps_output  LeftPortType=input  RightPortType=output  PseudoPeriodic=off  Frequencies=[]  VectorFormat=1-D array  Unit=inherit  AffineConversion=off
  + : PMIOPort  Side=Left
  - : PMIOPort  Port=2  Side=Right
  i : Outport
  wires:
  PS-Simulink Converter1/1 -> i/1
  connections:
  Current Sensor/RConn1 -- PS-Simulink Converter1/LConn1
  Current Sensor/LConn1 -- +/RConn1
  Current Sensor/RConn2 -- -/RConn1

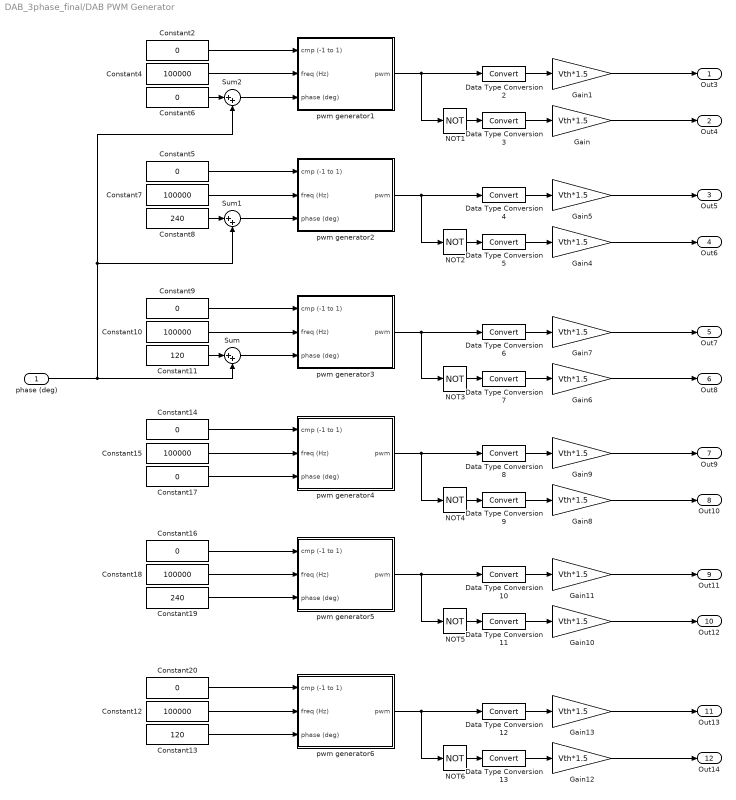
== system DAB_3phase_final/DAB PWM Generator ==
  phase (deg) : Inport
  Constant{4,7,10,12,15,18} (6 alike) : Constant  Value=100000
  Constant11 : Constant  Value=120
  Constant13 : Constant  Value=120
  Constant{2,5..6,9,14,16..17,20} (8 alike) : Constant  Value=0
  Constant19 : Constant  Value=240
  Constant8 : Constant  Value=240
  Data Type Conversion{2..13} (12 alike) : DataTypeConversion  SaturateOnIntegerOverflow=off  RndMeth=Floor
  Gain{,1,4..13} (12 alike) : Gain  Gain=Vth*1.5
  NOT{1..6} (6 alike) : Logic  Operator=NOT  IconShape=distinctive  AllPortsSameDT=off  OutDataTypeStr=boolean
  Sum : Sum  Inputs=|++
  Sum1 : Sum  Inputs=|++
  Sum2 : Sum  Inputs=|++
  pwm generator1 : Subsystem
  pwm generator2 : Subsystem
  pwm generator3 : Subsystem
  pwm generator4 : Subsystem
  pwm generator5 : Subsystem
  pwm generator6 : Subsystem
  Out3 : Outport
  Out4 : Outport  Port=2
  Out5 : Outport  Port=3
  Out6 : Outport  Port=4
  Out7 : Outport  Port=5
  Out8 : Outport  Port=6
  Out9 : Outport  Port=7
  Out10 : Outport  Port=8
  Out11 : Outport  Port=9
  Out12 : Outport  Port=10
  Out13 : Outport  Port=11
  Out14 : Outport  Port=12
  wires:
  NOT1/1 -> Data Type Conversion3/1
  pwm generator1/1(pwm) -> NOT1/1, Data Type Conversion2/1
  Constant2/1 -> pwm generator1/1(cmp (-1 to 1))
  Data Type Conversion2/1 -> Gain1/1
  Gain/1 -> Out4/1
  Data Type Conversion3/1 -> Gain/1
  Constant4/1 -> pwm generator1/2(freq (Hz))
  Gain1/1 -> Out3/1
  pwm generator2/1(pwm) -> NOT2/1, Data Type Conversion4/1
  Gain4/1 -> Out6/1
  Constant7/1 -> pwm generator2/2(freq (Hz))
  Constant5/1 -> pwm generator2/1(cmp (-1 to 1))
  Data Type Conversion5/1 -> Gain4/1
  Gain5/1 -> Out5/1
  Data Type Conversion4/1 -> Gain5/1
  NOT2/1 -> Data Type Conversion5/1
  Constant10/1 -> pwm generator3/2(freq (Hz))
  pwm generator3/1(pwm) -> NOT3/1, Data Type Conversion6/1
  Gain6/1 -> Out8/1
  Constant9/1 -> pwm generator3/1(cmp (-1 to 1))
  Data Type Conversion6/1 -> Gain7/1
  Gain7/1 -> Out7/1
  Data Type Conversion7/1 -> Gain6/1
  NOT3/1 -> Data Type Conversion7/1
  pwm generator5/1(pwm) -> NOT5/1, Data Type Conversion10/1
  Constant16/1 -> pwm generator5/1(cmp (-1 to 1))
  Gain12/1 -> Out14/1
  Constant20/1 -> pwm generator6/1(cmp (-1 to 1))
  Constant12/1 -> pwm generator6/2(freq (Hz))
  Gain10/1 -> Out12/1
  Constant13/1 -> pwm generator6/3(phase (deg))
  pwm generator4/1(pwm) -> NOT4/1, Data Type Conversion8/1
  Constant17/1 -> pwm generator4/3(phase (deg))
  Constant18/1 -> pwm generator5/2(freq (Hz))
  Data Type Conversion9/1 -> Gain8/1
  Gain9/1 -> Out9/1
  Gain8/1 -> Out10/1
  Constant19/1 -> pwm generator5/3(phase (deg))
  Data Type Conversion8/1 -> Gain9/1
  Constant15/1 -> pwm generator4/2(freq (Hz))
  Constant14/1 -> pwm generator4/1(cmp (-1 to 1))
  pwm generator6/1(pwm) -> NOT6/1, Data Type Conversion12/1
  Data Type Conversion10/1 -> Gain11/1
  Gain11/1 -> Out11/1
  Data Type Conversion13/1 -> Gain12/1
  NOT4/1 -> Data Type Conversion9/1
  NOT6/1 -> Data Type Conversion13/1
  Data Type Conversion11/1 -> Gain10/1
  NOT5/1 -> Data Type Conversion11/1
  Gain13/1 -> Out13/1
  Data Type Conversion12/1 -> Gain13/1
  Constant11/1 -> Sum/1
  Sum/1 -> pwm generator3/3(phase (deg))
  phase (deg)/1 -> Sum2/2, Sum1/2, Sum/2
  Constant8/1 -> Sum1/1
  Sum1/1 -> pwm generator2/3(phase (deg))
  Constant6/1 -> Sum2/1
  Sum2/1 -> pwm generator1/3(phase (deg))

== system DAB_3phase_final/Subsystem ==
  PS-Simulink Converter : nesl_utility/PS-Simulink Converter  PhysicalDomain=network_engine_domain  SubClassName=ps_output  LeftPortType=input  RightPortType=output  PseudoPeriodic=off  Frequencies=[]  VectorFormat=1-D array  Unit=inherit  AffineConversion=off
  Voltage Sensor : fl_lib/Electrical/Electrical Sensors/Voltage Sensor
  + : PMIOPort  Side=Left
  - : PMIOPort  Port=2  Side=Right
  v : Outport
  wires:
  PS-Simulink Converter/1 -> v/1
  connections:
  Voltage Sensor/LConn1 -- +/RConn1
  Voltage Sensor/RConn1 -- PS-Simulink Converter/LConn1
  Voltage Sensor/RConn2 -- -/RConn1

== system DAB_3phase_final/Subsystem1 ==
  PS-Simulink Converter : nesl_utility/PS-Simulink Converter  PhysicalDomain=network_engine_domain  SubClassName=ps_output  LeftPortType=input  RightPortType=output  PseudoPeriodic=off  Frequencies=[]  VectorFormat=1-D array  Unit=inherit  AffineConversion=off
  Voltage Sensor : fl_lib/Electrical/Electrical Sensors/Voltage Sensor
  + : PMIOPort  Side=Left
  - : PMIOPort  Port=2  Side=Right
  v : Outport
  wires:
  PS-Simulink Converter/1 -> v/1
  connections:
  Voltage Sensor/RConn2 -- -/RConn1
  Voltage Sensor/RConn1 -- PS-Simulink Converter/LConn1
  Voltage Sensor/LConn1 -- +/RConn1

== system DAB_3phase_final/Subsystem2 ==
  PS-Simulink Converter : nesl_utility/PS-Simulink Converter  PhysicalDomain=network_engine_domain  SubClassName=ps_output  LeftPortType=input  RightPortType=output  PseudoPeriodic=off  Frequencies=[]  VectorFormat=1-D array  Unit=inherit  AffineConversion=off
  Voltage Sensor : fl_lib/Electrical/Electrical Sensors/Voltage Sensor
  + : PMIOPort  Side=Left
  - : PMIOPort  Port=2  Side=Left
  v : Outport
  wires:
  PS-Simulink Converter/1 -> v/1
  connections:
  Voltage Sensor/RConn2 -- -/RConn1
  Voltage Sensor/RConn1 -- PS-Simulink Converter/LConn1
  Voltage Sensor/LConn1 -- +/RConn1

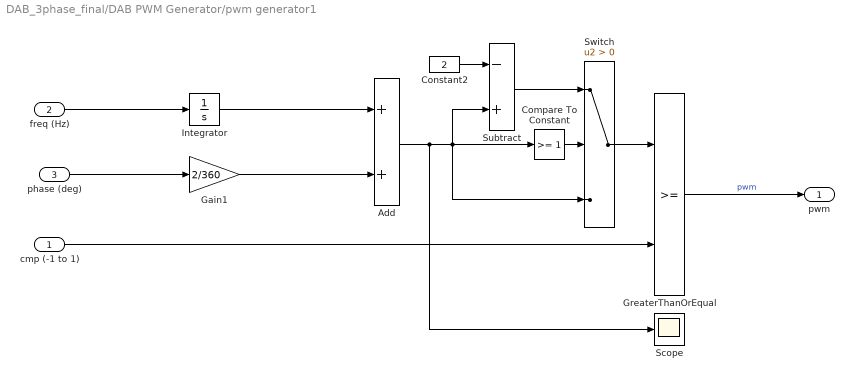
== system DAB_3phase_final/DAB PWM Generator/pwm generator1 ==
  cmp (-1 to 1) : Inport
  freq (Hz) : Inport  Port=2
  phase (deg) : Inport  Port=3
  Add : Sum
  Compare To Constant : simulink/Logic and Bit Operations/Compare To Constant  relop=>=  const=1  OutDataTypeStr=boolean
  Constant2 : Constant  Value=2
  Gain1 : Gain  Gain=2/360
  GreaterThanOrEqual : RelationalOperator  OutDataTypeStr=boolean  RndMeth=Simplest  InputSameDT=off
  Integrator : Integrator  WrapState=on  WrappedStateUpperValue=1  WrappedStateLowerValue=-1
  Scope : Scope
  Subtract : Sum  Inputs=-+
  Switch : Switch  Criteria=u2 > Threshold  SaturateOnIntegerOverflow=off  InputSameDT=off
  pwm : Outport
  wires:
  GreaterThanOrEqual/1 -> pwm/1  "pwm"
  phase (deg)/1 -> Gain1/1
  Switch/1 -> GreaterThanOrEqual/1
  Subtract/1 -> Switch/1
  Compare To Constant/1 -> Switch/2
  Integrator/1 -> Add/1
  Add/1 -> Scope/1, Compare To Constant/1, Subtract/2, Switch/3
  cmp (-1 to 1)/1 -> GreaterThanOrEqual/2
  freq (Hz)/1 -> Integrator/1
  Gain1/1 -> Add/2
  Constant2/1 -> Subtract/1

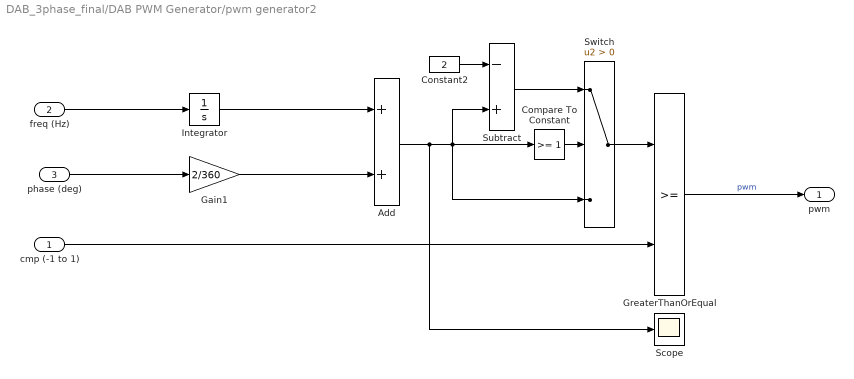
== system DAB_3phase_final/DAB PWM Generator/pwm generator2 ==
  cmp (-1 to 1) : Inport
  freq (Hz) : Inport  Port=2
  phase (deg) : Inport  Port=3
  Add : Sum
  Compare To Constant : simulink/Logic and Bit Operations/Compare To Constant  relop=>=  const=1  OutDataTypeStr=boolean
  Constant2 : Constant  Value=2
  Gain1 : Gain  Gain=2/360
  GreaterThanOrEqual : RelationalOperator  OutDataTypeStr=boolean  RndMeth=Simplest  InputSameDT=off
  Integrator : Integrator  WrapState=on  WrappedStateUpperValue=1  WrappedStateLowerValue=-1
  Scope : Scope
  Subtract : Sum  Inputs=-+
  Switch : Switch  Criteria=u2 > Threshold  SaturateOnIntegerOverflow=off  InputSameDT=off
  pwm : Outport
  wires:
  GreaterThanOrEqual/1 -> pwm/1  "pwm"
  phase (deg)/1 -> Gain1/1
  Switch/1 -> GreaterThanOrEqual/1
  Subtract/1 -> Switch/1
  Compare To Constant/1 -> Switch/2
  Integrator/1 -> Add/1
  Add/1 -> Scope/1, Compare To Constant/1, Subtract/2, Switch/3
  cmp (-1 to 1)/1 -> GreaterThanOrEqual/2
  freq (Hz)/1 -> Integrator/1
  Gain1/1 -> Add/2
  Constant2/1 -> Subtract/1

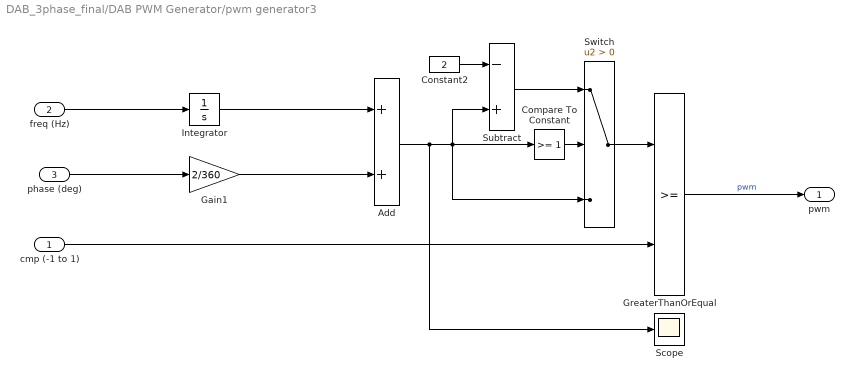
== system DAB_3phase_final/DAB PWM Generator/pwm generator3 ==
  cmp (-1 to 1) : Inport
  freq (Hz) : Inport  Port=2
  phase (deg) : Inport  Port=3
  Add : Sum
  Compare To Constant : simulink/Logic and Bit Operations/Compare To Constant  relop=>=  const=1  OutDataTypeStr=boolean
  Constant2 : Constant  Value=2
  Gain1 : Gain  Gain=2/360
  GreaterThanOrEqual : RelationalOperator  OutDataTypeStr=boolean  RndMeth=Simplest  InputSameDT=off
  Integrator : Integrator  WrapState=on  WrappedStateUpperValue=1  WrappedStateLowerValue=-1
  Scope : Scope
  Subtract : Sum  Inputs=-+
  Switch : Switch  Criteria=u2 > Threshold  SaturateOnIntegerOverflow=off  InputSameDT=off
  pwm : Outport
  wires:
  GreaterThanOrEqual/1 -> pwm/1  "pwm"
  phase (deg)/1 -> Gain1/1
  Switch/1 -> GreaterThanOrEqual/1
  Subtract/1 -> Switch/1
  Compare To Constant/1 -> Switch/2
  Integrator/1 -> Add/1
  Add/1 -> Scope/1, Compare To Constant/1, Subtract/2, Switch/3
  cmp (-1 to 1)/1 -> GreaterThanOrEqual/2
  freq (Hz)/1 -> Integrator/1
  Gain1/1 -> Add/2
  Constant2/1 -> Subtract/1

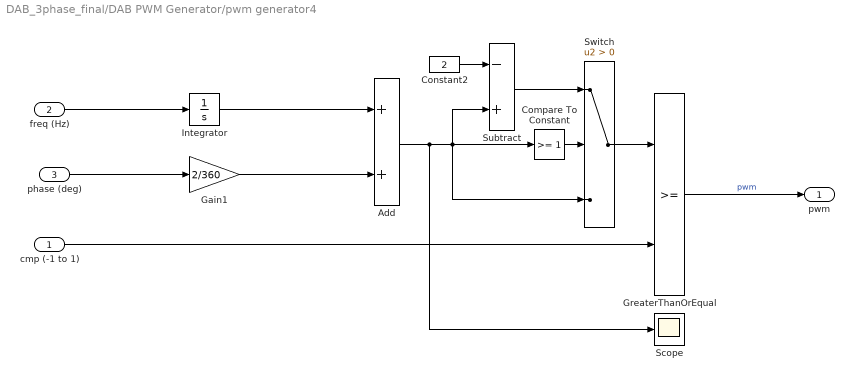
== system DAB_3phase_final/DAB PWM Generator/pwm generator4 ==
  cmp (-1 to 1) : Inport
  freq (Hz) : Inport  Port=2
  phase (deg) : Inport  Port=3
  Add : Sum
  Compare To Constant : simulink/Logic and Bit Operations/Compare To Constant  relop=>=  const=1  OutDataTypeStr=boolean
  Constant2 : Constant  Value=2
  Gain1 : Gain  Gain=2/360
  GreaterThanOrEqual : RelationalOperator  OutDataTypeStr=boolean  RndMeth=Simplest  InputSameDT=off
  Integrator : Integrator  WrapState=on  WrappedStateUpperValue=1  WrappedStateLowerValue=-1
  Scope : Scope
  Subtract : Sum  Inputs=-+
  Switch : Switch  Criteria=u2 > Threshold  SaturateOnIntegerOverflow=off  InputSameDT=off
  pwm : Outport
  wires:
  GreaterThanOrEqual/1 -> pwm/1  "pwm"
  phase (deg)/1 -> Gain1/1
  Switch/1 -> GreaterThanOrEqual/1
  Subtract/1 -> Switch/1
  Compare To Constant/1 -> Switch/2
  Integrator/1 -> Add/1
  Add/1 -> Scope/1, Compare To Constant/1, Subtract/2, Switch/3
  cmp (-1 to 1)/1 -> GreaterThanOrEqual/2
  freq (Hz)/1 -> Integrator/1
  Gain1/1 -> Add/2
  Constant2/1 -> Subtract/1

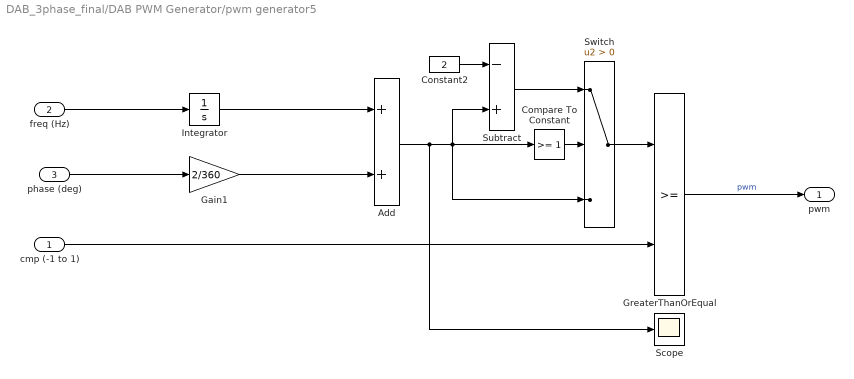
== system DAB_3phase_final/DAB PWM Generator/pwm generator5 ==
  cmp (-1 to 1) : Inport
  freq (Hz) : Inport  Port=2
  phase (deg) : Inport  Port=3
  Add : Sum
  Compare To Constant : simulink/Logic and Bit Operations/Compare To Constant  relop=>=  const=1  OutDataTypeStr=boolean
  Constant2 : Constant  Value=2
  Gain1 : Gain  Gain=2/360
  GreaterThanOrEqual : RelationalOperator  OutDataTypeStr=boolean  RndMeth=Simplest  InputSameDT=off
  Integrator : Integrator  WrapState=on  WrappedStateUpperValue=1  WrappedStateLowerValue=-1
  Scope : Scope
  Subtract : Sum  Inputs=-+
  Switch : Switch  Criteria=u2 > Threshold  SaturateOnIntegerOverflow=off  InputSameDT=off
  pwm : Outport
  wires:
  GreaterThanOrEqual/1 -> pwm/1  "pwm"
  phase (deg)/1 -> Gain1/1
  Switch/1 -> GreaterThanOrEqual/1
  Subtract/1 -> Switch/1
  Compare To Constant/1 -> Switch/2
  Integrator/1 -> Add/1
  Add/1 -> Scope/1, Compare To Constant/1, Subtract/2, Switch/3
  cmp (-1 to 1)/1 -> GreaterThanOrEqual/2
  freq (Hz)/1 -> Integrator/1
  Gain1/1 -> Add/2
  Constant2/1 -> Subtract/1

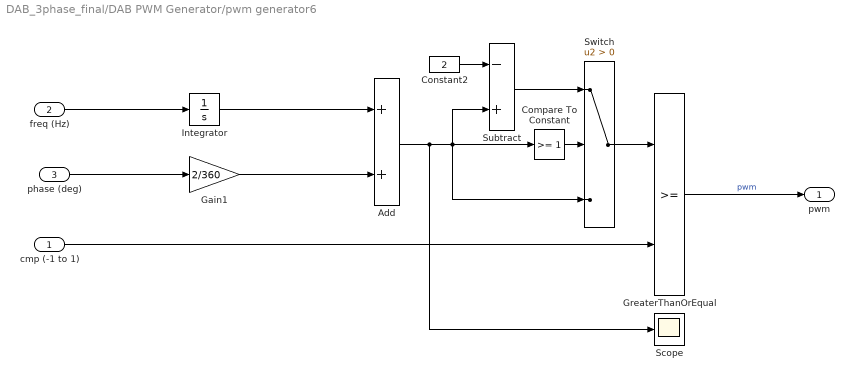
== system DAB_3phase_final/DAB PWM Generator/pwm generator6 ==
  cmp (-1 to 1) : Inport
  freq (Hz) : Inport  Port=2
  phase (deg) : Inport  Port=3
  Add : Sum
  Compare To Constant : simulink/Logic and Bit Operations/Compare To Constant  relop=>=  const=1  OutDataTypeStr=boolean
  Constant2 : Constant  Value=2
  Gain1 : Gain  Gain=2/360
  GreaterThanOrEqual : RelationalOperator  OutDataTypeStr=boolean  RndMeth=Simplest  InputSameDT=off
  Integrator : Integrator  WrapState=on  WrappedStateUpperValue=1  WrappedStateLowerValue=-1
  Scope : Scope
  Subtract : Sum  Inputs=-+
  Switch : Switch  Criteria=u2 > Threshold  SaturateOnIntegerOverflow=off  InputSameDT=off
  pwm : Outport
  wires:
  GreaterThanOrEqual/1 -> pwm/1  "pwm"
  phase (deg)/1 -> Gain1/1
  Switch/1 -> GreaterThanOrEqual/1
  Subtract/1 -> Switch/1
  Compare To Constant/1 -> Switch/2
  Integrator/1 -> Add/1
  Add/1 -> Scope/1, Compare To Constant/1, Subtract/2, Switch/3
  cmp (-1 to 1)/1 -> GreaterThanOrEqual/2
  freq (Hz)/1 -> Integrator/1
  Gain1/1 -> Add/2
  Constant2/1 -> Subtract/1
